simulink model "ContinuousIntegralAct"  (R2020b)
settings: Solver=FixedStepAuto  StartTime=0.0  StopTime=3  FixedStep=1e-4  RelTol=1e-4
undefined symbols (not defined in the file or in its folder): daq, drv, gbox, mech, mld, mot, rads2rpm, robust, rpm2rads, sens, state_space
settings Model: Creator=Utente  LastModifiedBy=Utente

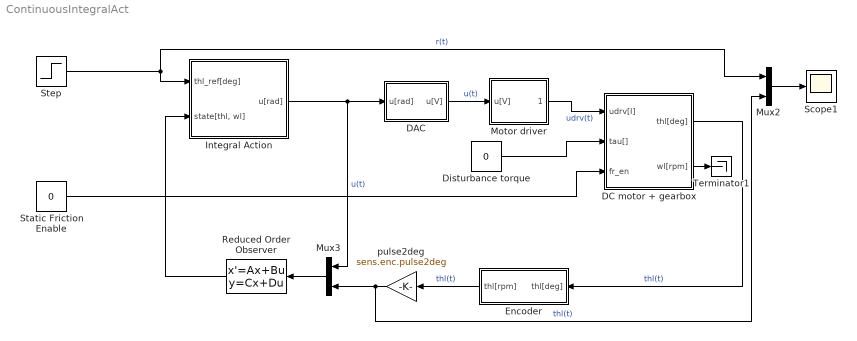
== system ContinuousIntegralAct ==
  DAC : Subsystem
  DC motor + gearbox : Subsystem
  Disturbance torque : Constant  Value=0
  Encoder : Subsystem
  Integral Action : Subsystem
  Motor driver : Subsystem
  Mux2 : Mux  Inputs=2
  Mux3 : Mux  Inputs=2
  Reduced Order Observer : StateSpace  A=state_space.A0  B=state_space.B0  C=state_space.C0  D=state_space.D0  InitialCondition=0
  Scope1 : Scope
  Static Friction Enable : Constant  Value=0
  Step : Step  Time=0  After=40  SampleTime=0
  Terminator1 : Terminator
  pulse2deg : Gain  Gain=sens.enc.pulse2deg
  wires:
  Motor driver/1(udrv[I]) -> DC motor + gearbox/1(udrv[I])  "udrv(t)"
  Static Friction Enable/1 -> DC motor + gearbox/3(fr_en)
  Reduced Order Observer/1 -> Integral Action/2("state[thl, wl]")
  Mux3/1 -> Reduced Order Observer/1
  Step/1 -> Integral Action/1(thl_ref[deg]), Mux2/1  "r(t)"
  Disturbance torque/1 -> DC motor + gearbox/2(tau[])
  Mux2/1 -> Scope1/1
  DAC/1(u[V]) -> Motor driver/1(u[V])  "u(t)"
  pulse2deg/1 -> Mux2/2, Mux3/2  "thl(t)"
  DC motor + gearbox/2(wl[rpm]) -> Terminator1/1
  Encoder/1(thl[rpm]) -> pulse2deg/1  "thl(t)"
  Integral Action/1(u[rad]) -> DAC/1(u[rad]), Mux3/1  "u(t)"
  DC motor + gearbox/1(thl[deg]) -> Encoder/1(thl[deg])  "thl(t)"

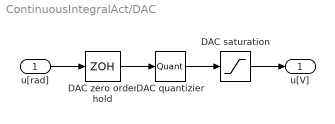
== system ContinuousIntegralAct/DAC ==
  u[rad] : Inport
  DAC quantizier : Quantizer  QuantizationInterval=daq.dac.q
  DAC saturation : Saturate  UpperLimit=daq.dac.vdd  LowerLimit=daq.dac.vss
  DAC zero order hold : ZeroOrderHold  SampleTime=daq.dac.T_s
  u[V] : Outport
  wires:
  DAC quantizier/1 -> DAC saturation/1
  DAC zero order hold/1 -> DAC quantizier/1
  DAC saturation/1 -> u[V]/1
  u[rad]/1 -> DAC zero order hold/1

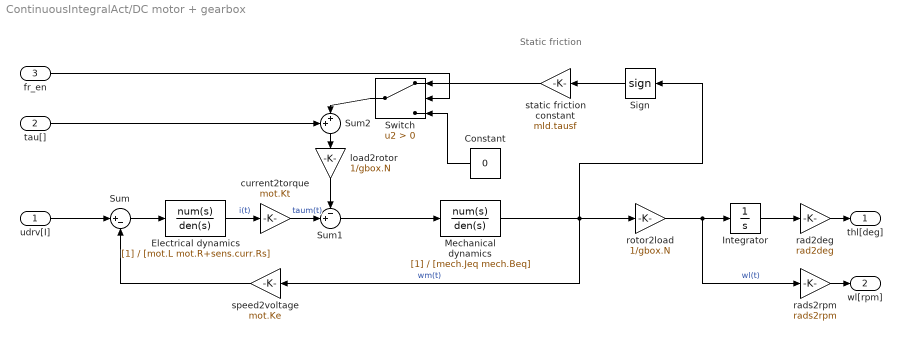
== system ContinuousIntegralAct/DC motor + gearbox ==
  note: Static friction
  udrv[I] : Inport  Unit=V
  tau[] : Inport  Port=2  Unit=V
  fr_en : Inport  Port=3  Unit=V
  Constant : Constant  Value=0
  Electrical dynamics : TransferFcn  Denominator=[mot.L mot.R+sens.curr.Rs]
  Integrator : Integrator
  Mechanical dynamics : TransferFcn  Denominator=[mech.Jeq mech.Beq]
  Sign : Signum  ZeroCross=off
  Sum : Sum  Inputs=|+-
  Sum1 : Sum  Inputs=-+|
  Sum2 : Sum  Inputs=++|
  Switch : Switch  Criteria=u2 > Threshold
  current2torque : Gain  Gain=mot.Kt
  load2rotor : Gain  Gain=1/gbox.N
  rad2deg : Gain  Gain=rad2deg
  rads2rpm : Gain  Gain=rads2rpm
  rotor2load : Gain  Gain=1/gbox.N
  speed2voltage : Gain  Gain=mot.Ke
  static friction constant : Gain  Gain=mld.tausf
  thl[deg] : Outport  Unit=deg
  wl[rpm] : Outport  Port=2  Unit=rpm
  wires:
  load2rotor/1 -> Sum1/1
  Mechanical dynamics/1 -> Sign/1, rotor2load/1, speed2voltage/1  "wm(t)"
  Sign/1 -> static friction constant/1
  current2torque/1 -> Sum1/2  "taum(t)"
  Sum1/1 -> Mechanical dynamics/1
  speed2voltage/1 -> Sum/2
  rotor2load/1 -> rads2rpm/1, Integrator/1  "wl(t)"
  Electrical dynamics/1 -> current2torque/1  "i(t)"
  Integrator/1 -> rad2deg/1
  Sum/1 -> Electrical dynamics/1
  rads2rpm/1 -> wl[rpm]/1
  rad2deg/1 -> thl[deg]/1
  udrv[I]/1 -> Sum/1
  Sum2/1 -> load2rotor/1
  tau[]/1 -> Sum2/1
  static friction constant/1 -> Switch/1
  Switch/1 -> Sum2/2
  Constant/1 -> Switch/3
  fr_en/1 -> Switch/2

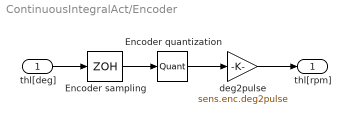
== system ContinuousIntegralAct/Encoder ==
  thl[deg] : Inport
  Encoder quantization : Quantizer  QuantizationInterval=sens.enc.q
  Encoder sampling : ZeroOrderHold  SampleTime=sens.enc.T_s
  deg2pulse : Gain  Gain=sens.enc.deg2pulse
  thl[rpm] : Outport
  wires:
  Encoder quantization/1 -> deg2pulse/1
  deg2pulse/1 -> thl[rpm]/1
  Encoder sampling/1 -> Encoder quantization/1
  thl[deg]/1 -> Encoder sampling/1

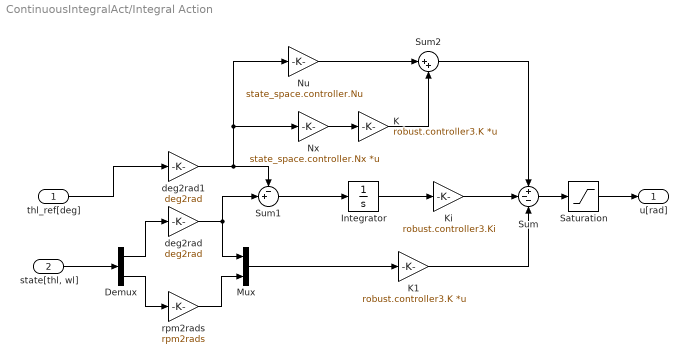
== system ContinuousIntegralAct/Integral Action ==
  thl_ref[deg] : Inport
  "state[thl, wl]" : Inport  Port=2
  Demux : Demux  Outputs=2
  Integrator : Integrator
  K : Gain  Gain=robust.controller3.K  Multiplication=Matrix(K*u)
  K1 : Gain  Gain=robust.controller3.K  Multiplication=Matrix(K*u)
  Ki : Gain  Gain=robust.controller3.Ki
  Mux : Mux  Inputs=2
  Nu : Gain  Gain=state_space.controller.Nu
  Nx : Gain  Gain=state_space.controller.Nx  Multiplication=Matrix(K*u)
  Saturation : Saturate  UpperLimit=daq.dac.vdd  LowerLimit=daq.dac.vss
  Sum : Sum  Inputs=+--
  Sum1 : Sum  Inputs=-+|
  Sum2 : Sum  Inputs=|++
  deg2rad : Gain  Gain=deg2rad
  deg2rad1 : Gain  Gain=deg2rad
  rpm2rads : Gain  Gain=rpm2rads
  u[rad] : Outport
  wires:
  Saturation/1 -> u[rad]/1
  "state[thl, wl]"/1 -> Demux/1
  Integrator/1 -> Ki/1
  Ki/1 -> Sum/2
  Demux/1 -> deg2rad/1
  thl_ref[deg]/1 -> deg2rad1/1
  Sum1/1 -> Integrator/1
  K1/1 -> Sum/3
  Sum/1 -> Saturation/1
  Mux/1 -> K1/1
  deg2rad/1 -> Mux/1, Sum1/2
  Demux/2 -> rpm2rads/1
  rpm2rads/1 -> Mux/2
  deg2rad1/1 -> Nx/1, Nu/1, Sum1/1
  Nu/1 -> Sum2/1
  Sum2/1 -> Sum/1
  Nx/1 -> K/1
  K/1 -> Sum2/2

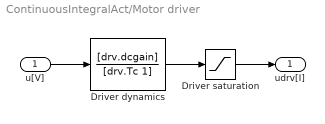
== system ContinuousIntegralAct/Motor driver ==
  u[V] : Inport
  Driver dynamics : TransferFcn  Numerator=[drv.dcgain]  Denominator=[drv.Tc 1]
  Driver saturation : Saturate  UpperLimit=drv.vp  LowerLimit=drv.vm
  udrv[I] : Outport
  wires:
  Driver saturation/1 -> udrv[I]/1
  Driver dynamics/1 -> Driver saturation/1
  u[V]/1 -> Driver dynamics/1
